simulink model "M_B_K_simulink"  (R2015a)
settings: Solver=ode8  StartTime=0.0  StopTime=200  FixedStep=0.0001  RelTol=1e-3
values from neighbouring files (symbols this model uses):
  B1 = 20    [Prac_5_Solution.m]
  B2 = 20    [Prac_5_Solution.m]
  B3 = 30    [Prac_5_Solution.m]
  f = 300    [Prac_5_Solution.m]
  K1 = 15    [Prac_5_Solution.m]
  K2 = 15    [Prac_5_Solution.m]
  M1 = 750    [Prac_5_Solution.m]
  M2 = 750    [Prac_5_Solution.m]
settings Model: Creator=DELL  LastModifiedBy=DELL

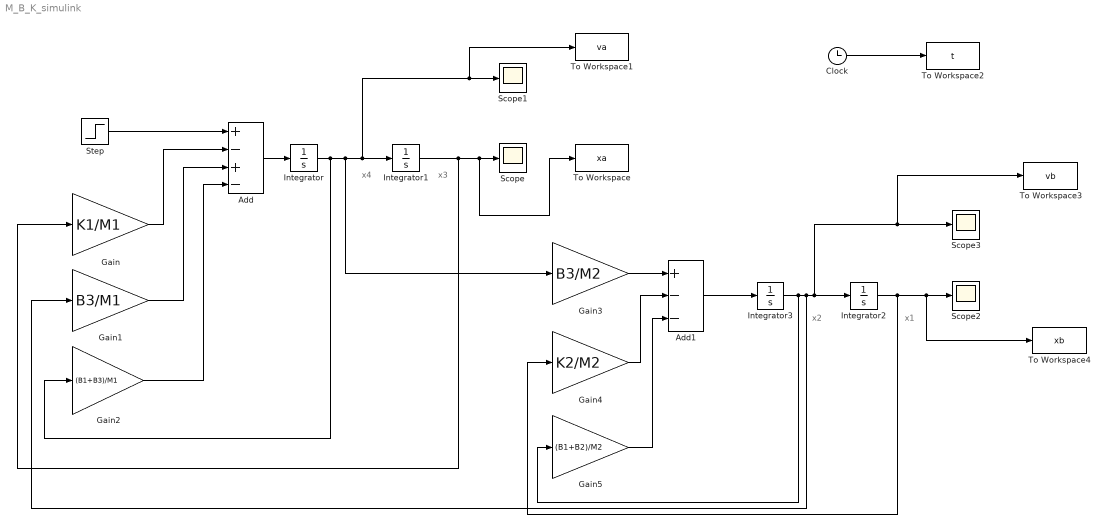
== system M_B_K_simulink ==
  note: x1
  note: x2
  note: x3
  note: x4
  Add : Sum  Inputs=+-+-
  Add1 : Sum  Inputs=+--
  Clock : Clock
  Gain : Gain  Gain=K1/M1
  Gain1 : Gain  Gain=B3/M1
  Gain2 : Gain  Gain=(B1+B3)/M1
  Gain3 : Gain  Gain=B3/M2
  Gain4 : Gain  Gain=K2/M2
  Gain5 : Gain  Gain=(B1+B2)/M2
  Integrator{,1..3} (4 alike) : Integrator
  Scope{,1..3} (4 alike) : Scope
      Scope2 settings: SaveName=ScopeData2
      Scope3 settings: SaveName=ScopeData3
  Step : Step  Time=0  After=f/M1  SampleTime=0
  To Workspace : ToWorkspace  VariableName=xa  SampleTime=-1
  To Workspace1 : ToWorkspace  VariableName=va  SampleTime=-1
  To Workspace2 : ToWorkspace  VariableName=t  SampleTime=-1
  To Workspace3 : ToWorkspace  VariableName=vb  SampleTime=-1
  To Workspace4 : ToWorkspace  VariableName=xb  SampleTime=-1
  wires:
  Integrator/1 -> Integrator1/1, Scope1/1, To Workspace1/1, Gain3/1, Gain2/1
  Integrator1/1 -> Scope/1, To Workspace/1, Gain/1
  Add/1 -> Integrator/1
  Step/1 -> Add/1
  Gain/1 -> Add/2
  Gain1/1 -> Add/3
  Clock/1 -> To Workspace2/1
  Gain2/1 -> Add/4
  Integrator3/1 -> Gain1/1, To Workspace3/1, Scope3/1, Integrator2/1, Gain5/1
  Integrator2/1 -> Gain4/1, Scope2/1, To Workspace4/1
  Add1/1 -> Integrator3/1
  Gain3/1 -> Add1/1
  Gain4/1 -> Add1/2
  Gain5/1 -> Add1/3
